simulink model "Sim40"  (R2019a)
settings: Solver=FixedStepAuto  StartTime=0.0  StopTime=10.0  FixedStep=0.0001  RelTol=1e-3
settings Model: Creator=fbleo  LastModifiedBy=fbleo

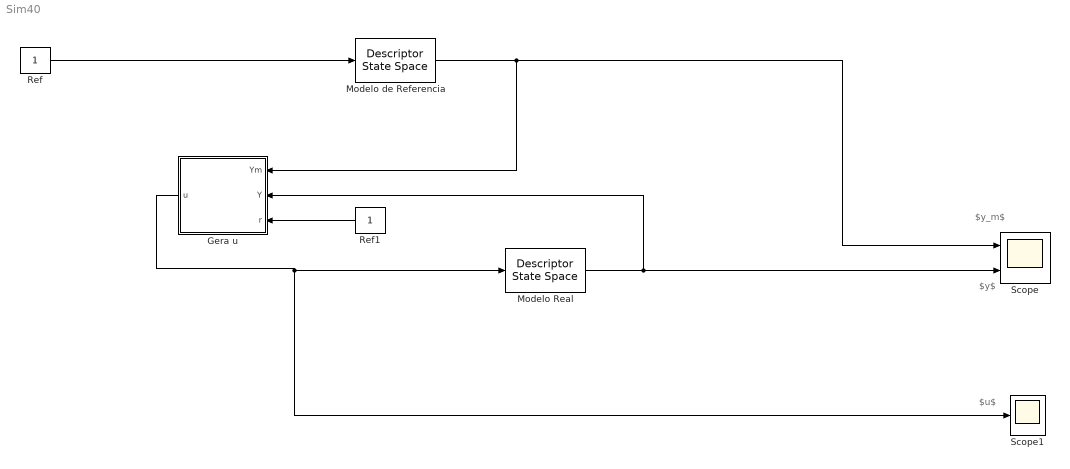
== system Sim40 ==
  note: $y$
  note: $u$
  note: $y_m$
  Gera u : Subsystem
  Modelo Real : DescriptorStateSpace  A=-1  B=2  D=0  InitialCondition=0.5
  Modelo de Referencia : DescriptorStateSpace  A=-3  B=3  D=0  InitialCondition=0
  Ref : Constant
  Ref1 : Constant
  Scope : Scope  NumInputPorts=2
  Scope1 : Scope
  wires:
  Modelo de Referencia/1 -> Scope/1, Gera u/1(Ym)
  Ref/1 -> Modelo de Referencia/1
  Gera u/1(u) -> Modelo Real/1, Scope1/1
  Modelo Real/1 -> Gera u/2(Y), Scope/2
  Ref1/1 -> Gera u/3(r)

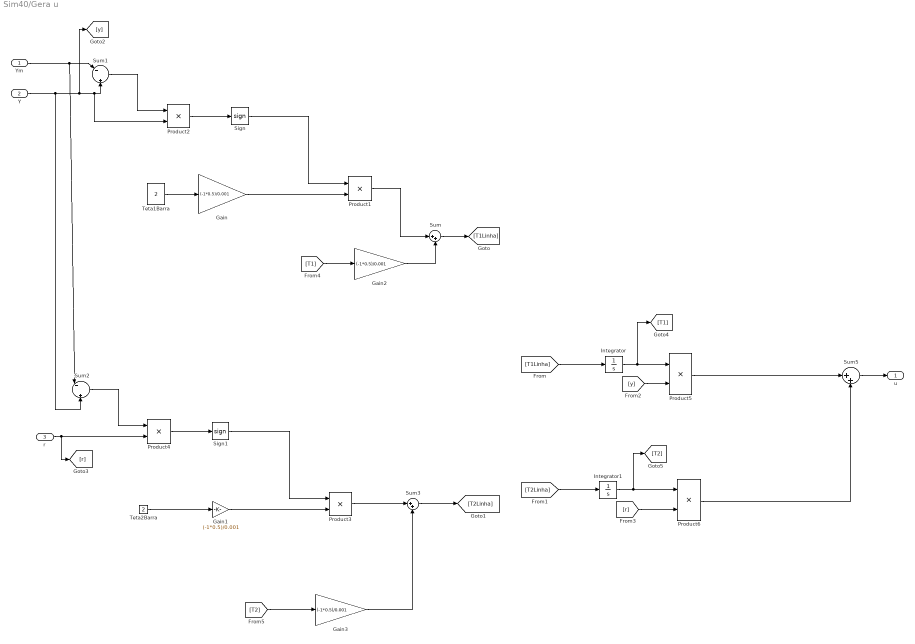
== system Sim40/Gera u ==
  Ym : Inport
  Y : Inport  Port=2
  r : Inport  Port=3
  Gain{,1..3} (4 alike) : Gain  Gain=(-1*0.5)/0.001
  Integrator : Integrator  InitialCondition=-0.65
  Integrator1 : Integrator  InitialCondition=1.14
  Product{1..6} (6 alike) : Product
  Sign : Signum
  Sign1 : Signum
  Sum : Sum  Inputs=|++
  Sum1 : Sum  Inputs=|-||+
  Sum2 : Sum  Inputs=|-||+
  Sum3 : Sum  Inputs=|++
  Sum5 : Sum  Inputs=|++
  Teta1Barra : Constant  Value=2
  Teta2Barra : Constant  Value=2
  u : Outport
  wires:
  Sign/1 -> Product1/1
  Gain/1 -> Product1/2
  Teta1Barra/1 -> Gain/1
  Sum1/1 -> Product2/1
  Product2/1 -> Sign/1
  Product1/1 -> Sum/1
  Ym/1 -> Sum1/1, Sum2/1
  Sign1/1 -> Product3/1
  Product4/1 -> Sign1/1
  Sum2/1 -> Product4/1
  Gain1/1 -> Product3/2
  Y/1 -> [y], Product2/2, Sum1/2, Sum2/2
  Teta2Barra/1 -> Gain1/1
  r/1 -> [r], Product4/2
  [y] -> Product5/2
  [T1Linha] -> Integrator/1
  [T2Linha] -> Integrator1/1
  [r] -> Product6/2
  Product5/1 -> Sum5/1
  Product6/1 -> Sum5/2
  Sum5/1 -> u/1
  Sum/1 -> [T1Linha]
  Integrator/1 -> [T1], Product5/1
  [T1] -> Gain2/1
  Gain2/1 -> Sum/2
  Integrator1/1 -> [T2], Product6/1
  Product3/1 -> Sum3/1
  Sum3/1 -> [T2Linha]
  [T2] -> Gain3/1
  Gain3/1 -> Sum3/2
